simulink model "LR_5_var2"  (R2020b)
settings: Solver=VariableStepAuto  StartTime=0.0  StopTime=5  FixedStep=1e-4  RelTol=1e-3
values from neighbouring files (symbols this model uses):
  a = 0.2    [LR_5_param_var2.m]
  b = 1.5    [LR_5_param_var2.m]
  c1 = 4    [LR_5_param_var2.m]
  U = 3    [LR_5_param_var2.m]
  w = 10    [LR_5_param_var2.m]
libraries: simulink x17, powerlib_meascontrol x6
settings Model: SimulationMode=accelerator  Creator=SIA  LastModifiedBy=SIA
settings SolverCC: ZeroCrossAlgorithm=Adaptive  AlgebraicLoopSolver=LineSearch
settings DebuggingCC: IgnoredZcDiagnostic=none

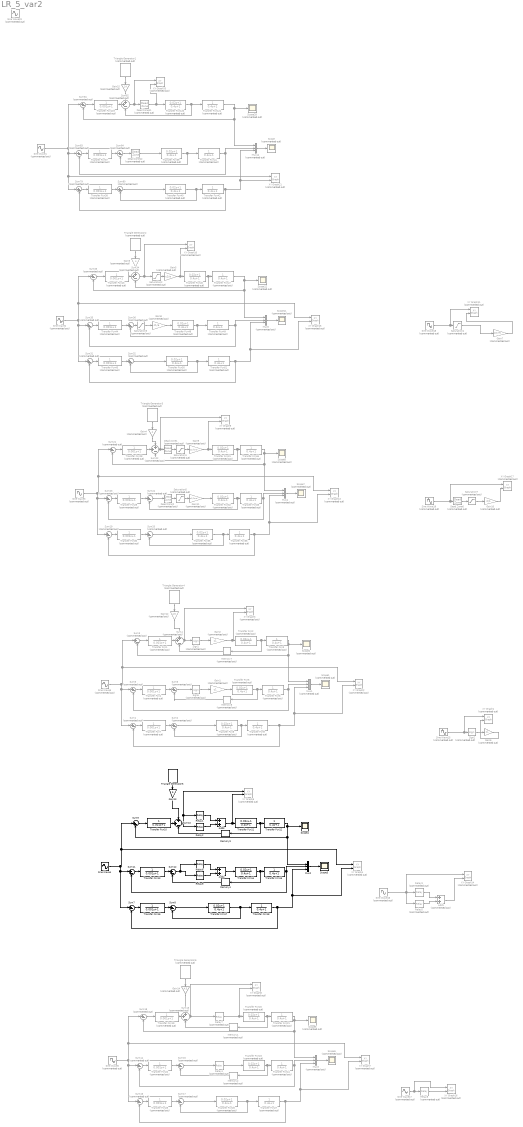
== system LR_5_var2 ==
  Add1 : Sum  Commented=on
  Add3 : Sum
  Add4 : Sum
  Dead Zone{1..2,11..12} (4 alike) : DeadZone  Commented=on  LowerValue=-a  UpperValue=a  SaturateOnIntegerOverflow=on
  Dead Zone6 : DeadZone  Commented=on  LowerValue=-1  UpperValue=1  SaturateOnIntegerOverflow=on
  Gain1 : Gain  Commented=on  Gain=c1
  Gain10 : Gain  Commented=on  Gain=2/1
  Gain11 : Gain  Commented=on  Gain=c1/(b-a)
  Gain12 : Gain  Commented=on  Gain=4.5
  Gain13 : Gain  Gain=5
  Gain14 : Gain  Commented=on  Gain=4.5
  Gain15 : Gain  Commented=on  Gain=14
  Gain2 : Gain  Commented=on  Gain=c1
  Gain3 : Gain  Commented=on  Gain=4
  Gain4 : Gain  Commented=on  Gain=4
  Gain5 : Gain  Commented=on  Gain=c1/a
  Gain6 : Gain  Commented=on  Gain=c1
  Gain7 : Gain  Commented=on  Gain=2/0.75
  Gain8 : Gain  Commented=on  Gain=c1/a
  Gain9 : Gain  Commented=on  Gain=c1/(b-a)
  Memory{1..2,7..8} (4 alike) : Memory  Commented=on
  Memory3 : Memory
  Memory4 : Memory
  Mux{1,3..4,6,14} (5 alike) : Mux  Commented=on  Inputs=3
  Mux2 : Mux  Inputs=3
  Relay1 : Relay  OnSwitchValue=a  OffSwitchValue=a  OnOutputValue=c1
  Relay2 : Relay  OnSwitchValue=-a  OffSwitchValue=-a  OnOutputValue=0  OffOutputValue=-c1
  Relay3 : Relay  Commented=on  OnSwitchValue=a  OffSwitchValue=a  OnOutputValue=c1
  Relay4 : Relay  Commented=on  OnSwitchValue=a  OffSwitchValue=-a  OnOutputValue=c1  OffOutputValue=-c1
  Relay5 : Relay  Commented=on  OnSwitchValue=-a  OffSwitchValue=-a  OnOutputValue=0  OffOutputValue=-c1
  Relay6 : Relay  OnSwitchValue=a  OffSwitchValue=a  OnOutputValue=c1
  Relay7 : Relay  Commented=on  OnSwitchValue=a  OffSwitchValue=-a  OnOutputValue=c1  OffOutputValue=-c1
  Relay8 : Relay  Commented=on  OnSwitchValue=a  OffSwitchValue=-a  OnOutputValue=c1  OffOutputValue=-c1
  Relay9 : Relay  OnSwitchValue=-a  OffSwitchValue=-a  OnOutputValue=0  OffOutputValue=-c1
  Saturation1 : Saturate  Commented=on  UpperLimit=b-a  LowerLimit=-(b-a)
  Saturation2 : Saturate  Commented=on  UpperLimit=a  LowerLimit=-a
  Saturation3 : Saturate  Commented=on  UpperLimit=a  LowerLimit=-a
  Saturation4 : Saturate  Commented=on  UpperLimit=0.75  LowerLimit=-0.75
  Saturation5 : Saturate  Commented=on  UpperLimit=b-a  LowerLimit=-(b-a)
  Saturation7 : Saturate  Commented=on  UpperLimit=1  LowerLimit=-1
  Scope{,1..2,5..8,11..12,28} (10 alike) : Scope  Commented=on
  Scope3 : Scope
  Scope4 : Scope
  Sign1 : Signum  Commented=on
  Sign2 : Signum  Commented=on
  Sign5 : Signum  Commented=on
  Sine Wave{1..3,5..6} (5 alike) : Sin  Commented=on  Amplitude=U  Frequency=w  SampleTime=0
  Sine Wave15 : Sin  Commented=on  Amplitude=3  Frequency=10  SampleTime=0
  Sine Wave16 : Sin  Commented=on  Amplitude=3  Phase=90  SampleTime=0
  Sine Wave17 : Sin  Commented=on  Amplitude=10  SampleTime=0
  Sine Wave18 : Sin  Commented=on  Amplitude=3  SampleTime=0
  Sine Wave19 : Sin  Commented=on  Amplitude=5  SampleTime=0
  Sine Wave23 : Sin  Commented=on  Amplitude=6  Frequency=1000  SampleTime=0
  Sine Wave4 : Sin  Amplitude=U  Frequency=w  SampleTime=0
  Sum{1..3,5..6,14..21,23..24,31..33,35..36,79..81,83..84} (25 alike) : Sum  Commented=on  Inputs=|+-
  Sum10 : Sum  Inputs=++-
  Sum{7..9,11..12} (5 alike) : Sum  Inputs=|+-
  Sum{4,13,22,34,82} (5 alike) : Sum  Commented=on  Inputs=++-
  Transfer Fcn{1,4,7,19,22,25,28..30,37..38,43..45,119} (15 alike) : TransferFcn  Commented=on  Denominator=[0.001 1]
  Transfer Fcn10 : TransferFcn  Denominator=[0.001 1]
  Transfer Fcn11 : TransferFcn  Numerator=[0.02 1]  Denominator=[0.4 1]
  Transfer Fcn12 : TransferFcn  Denominator=[0.4 1]
  Transfer Fcn{2,5,8,20,23,26,31..32,35,39..40,46,48,50,120} (15 alike) : TransferFcn  Commented=on  Numerator=[0.02 1]  Denominator=[0.4 1]
  Transfer Fcn{3,6,9,21,24,27,33..34,36,41..42,47,49,51,121} (15 alike) : TransferFcn  Commented=on  Denominator=[0.4 1]
  Transfer Fcn13 : TransferFcn  Denominator=[0.001 1]
  Transfer Fcn14 : TransferFcn  Numerator=[0.02 1]  Denominator=[0.4 1]
  Transfer Fcn15 : TransferFcn  Denominator=[0.4 1]
  Transfer Fcn16 : TransferFcn  Denominator=[0.001 1]
  Transfer Fcn17 : TransferFcn  Numerator=[0.02 1]  Denominator=[0.4 1]
  Transfer Fcn18 : TransferFcn  Denominator=[0.4 1]
  Triangle Generator{1..4} (4 alike) : powerlib_meascontrol/Pulse & Signal Generators/Triangle Generator  Commented=on  Freq=159.15494327  Phase=0  Ts=0
  Triangle Generator5 : powerlib_meascontrol/Pulse & Signal Generators/Triangle Generator  Freq=159.15494327  Phase=0  Ts=0
  Triangle Generator6 : powerlib_meascontrol/Pulse & Signal Generators/Triangle Generator  Commented=on  Freq=1590.15494327  Phase=0  Ts=0
  XY Graph1 : simulink/Sinks/XY Graph  Commented=on  xmin=-1  xmax=1  ymin=-4  ymax=4  st=0.001
  XY Graph10 : simulink/Sinks/XY Graph  Commented=on  xmin=-2  xmax=2  ymin=-4  ymax=4  st=-1
  XY Graph11 : simulink/Sinks/XY Graph  Commented=on  xmin=-1  xmax=1  ymin=-2  ymax=2  st=0.001
  XY Graph{2,4,7,13} (4 alike) : simulink/Sinks/XY Graph  Commented=on  xmin=-3  xmax=3  ymin=-0.5  ymax=0.5  st=0
  XY Graph14 : simulink/Sinks/XY Graph  Commented=on  xmin=-2  xmax=2  ymin=-4  ymax=4  st=0.001
  XY Graph15 : simulink/Sinks/XY Graph  Commented=on  xmin=-10  xmax=10  ymin=-0.3  ymax=0.3  st=0
  XY Graph16 : simulink/Sinks/XY Graph  Commented=on  xmin=-2  xmax=2  ymin=-4  ymax=4  st=0.001
  XY Graph17 : simulink/Sinks/XY Graph  Commented=on  xmin=-4  xmax=4  ymin=-2  ymax=2  st=0.001
  XY Graph20 : simulink/Sinks/XY Graph  Commented=on  xmin=-2  xmax=2  ymin=-1  ymax=1  st=-1
  XY Graph21 : simulink/Sinks/XY Graph  Commented=on  xmin=-10  xmax=10  ymin=-0.3  ymax=0.3  st=0
  XY Graph3 : simulink/Sinks/XY Graph  Commented=on  xmin=-2  xmax=2  ymin=-3  ymax=3  st=-1
  XY Graph6 : simulink/Sinks/XY Graph  Commented=on  xmin=-2  xmax=2  ymin=-3  ymax=3  st=-1
  XY Graph8 : simulink/Sinks/XY Graph  Commented=on  xmin=-2  xmax=2  ymin=-3  ymax=3  st=-1
  XY Graph9 : simulink/Sinks/XY Graph  Commented=on  xmin=-2  xmax=2  ymin=-4  ymax=4  st=-1
  wires:
  Sine Wave15/1 -> XY Graph1/1, Sign2/1
  Sign2/1 -> Gain6/1
  Gain6/1 -> XY Graph1/2
  Sine Wave16/1 -> Relay5/1, Relay3/1, XY Graph14/1
  Sine Wave17/1 -> Relay8/1, XY Graph16/1
  Relay8/1 -> XY Graph16/2
  Gain7/1 -> XY Graph11/2
  Sine Wave18/1 -> Saturation4/1, XY Graph11/1
  Saturation4/1 -> Gain7/1
  Sine Wave19/1 -> Dead Zone6/1, XY Graph17/1
  Gain10/1 -> XY Graph17/2
  Saturation7/1 -> Gain10/1
  Dead Zone6/1 -> Saturation7/1
  Transfer Fcn42/1 -> XY Graph21/2, Mux14/3, Sum79/2
  Transfer Fcn40/1 -> Transfer Fcn42/1, Sum80/2
  Sum80/1 -> Transfer Fcn40/1
  Dead Zone12/1 -> Transfer Fcn39/1
  Transfer Fcn39/1 -> Transfer Fcn41/1, Sum84/2
  Transfer Fcn121/1 -> Scope28/1, Mux14/1, Sum81/2
  Transfer Fcn41/1 -> Sum83/2, Mux14/2
  Transfer Fcn119/1 -> Sum82/2
  Sum82/1 -> XY Graph20/1, Dead Zone11/1
  Transfer Fcn37/1 -> Sum84/1
  Sum81/1 -> Transfer Fcn119/1
  Transfer Fcn38/1 -> Sum80/1
  Sum84/1 -> Dead Zone12/1
  Mux14/1 -> Scope/1
  Sum83/1 -> Transfer Fcn37/1
  Transfer Fcn120/1 -> Sum82/3, Transfer Fcn121/1
  Dead Zone11/1 -> XY Graph20/2, Transfer Fcn120/1
  Sum79/1 -> Transfer Fcn38/1
  Sine Wave1/1 -> Sum81/1, Sum79/1, XY Graph21/1, Sum83/1
  Transfer Fcn44/1 -> Sum36/1
  Sum35/1 -> Transfer Fcn44/1
  Saturation3/1 -> Gain8/1
  Transfer Fcn50/1 -> Transfer Fcn51/1, Sum32/2
  Transfer Fcn47/1 -> Scope12/1, Mux6/1, Sum33/2
  Transfer Fcn46/1 -> Transfer Fcn47/1, Sum34/3
  Saturation2/1 -> Gain5/1
  Transfer Fcn48/1 -> Transfer Fcn49/1, Sum36/2
  Sum31/1 -> Transfer Fcn45/1
  Sine Wave2/1 -> Sum33/1, XY Graph15/1, Sum31/1, Sum35/1
  Sum32/1 -> Transfer Fcn50/1
  Sum36/1 -> Saturation3/1
  Sum33/1 -> Transfer Fcn43/1
  Sum34/1 -> Saturation2/1, XY Graph10/1
  Mux6/1 -> Scope11/1
  Transfer Fcn43/1 -> Sum34/2
  Transfer Fcn51/1 -> XY Graph15/2, Mux6/3, Sum31/2
  Transfer Fcn45/1 -> Sum32/1
  Transfer Fcn49/1 -> Sum35/2, Mux6/2
  Gain5/1 -> Transfer Fcn46/1, XY Graph10/2
  Gain8/1 -> Transfer Fcn48/1
  Gain11/1 -> Transfer Fcn32/1
  Transfer Fcn34/1 -> Scope8/1, Mux4/1, Sum21/2
  Transfer Fcn29/1 -> Sum24/1
  Sum23/1 -> Transfer Fcn29/1
  Sum19/1 -> Transfer Fcn30/1
  Transfer Fcn32/1 -> Transfer Fcn33/1, Sum24/2
  Transfer Fcn31/1 -> Transfer Fcn34/1, Sum22/3
  Sine Wave3/1 -> Sum21/1, XY Graph13/1, Sum19/1, Sum23/1
  Sum20/1 -> Transfer Fcn35/1
  Gain9/1 -> Transfer Fcn31/1, XY Graph9/2
  Transfer Fcn33/1 -> Sum23/2, Mux4/2
  Transfer Fcn35/1 -> Transfer Fcn36/1, Sum20/2
  Transfer Fcn36/1 -> XY Graph13/2, Mux4/3, Sum19/2
  Mux4/1 -> Scope7/1
  Sum22/1 -> Dead Zone1/1, XY Graph9/1
  Transfer Fcn30/1 -> Sum20/1
  Transfer Fcn28/1 -> Sum22/2
  Gain4/1 -> Sum22/1
  Sum24/1 -> Dead Zone2/1
  Sum21/1 -> Transfer Fcn28/1
  Dead Zone2/1 -> Saturation5/1
  Saturation5/1 -> Gain11/1
  Gain2/1 -> XY Graph3/2, Transfer Fcn2/1
  Transfer Fcn1/1 -> Sum4/2
  Transfer Fcn7/1 -> Sum2/1
  Sum4/1 -> Sign1/1, XY Graph3/1
  Sum3/1 -> Transfer Fcn1/1
  Mux1/1 -> Scope1/1
  Transfer Fcn9/1 -> XY Graph2/2, Mux1/3, Sum1/2
  Transfer Fcn6/1 -> Sum5/2, Mux1/2
  Sum2/1 -> Transfer Fcn8/1
  Transfer Fcn5/1 -> Transfer Fcn6/1, Memory8/1
  Transfer Fcn2/1 -> Transfer Fcn3/1, Memory7/1
  Transfer Fcn4/1 -> Sum6/1
  Sum1/1 -> Transfer Fcn7/1
  Transfer Fcn8/1 -> Transfer Fcn9/1, Sum2/2
  Sum5/1 -> Transfer Fcn4/1
  Gain1/1 -> Transfer Fcn5/1
  Sine Wave5/1 -> Sum3/1, XY Graph2/1, Sum1/1, Sum5/1
  Sum6/1 -> Sign5/1
  Transfer Fcn3/1 -> Scope2/1, Mux1/1, Sum3/2
  Sign1/1 -> Gain2/1
  Sign5/1 -> Gain1/1
  Memory7/1 -> Sum4/3
  Memory8/1 -> Sum6/2
  Add3/1 -> Transfer Fcn11/1, XY Graph6/2
  Sum9/1 -> Transfer Fcn10/1
  Transfer Fcn16/1 -> Sum8/1
  Memory4/1 -> Sum12/2
  Transfer Fcn14/1 -> Transfer Fcn15/1, Memory4/1
  Sum8/1 -> Transfer Fcn17/1
  Transfer Fcn10/1 -> Sum10/2
  Transfer Fcn13/1 -> Sum12/1
  Transfer Fcn18/1 -> XY Graph4/2, Mux2/3, Sum7/2
  Sine Wave4/1 -> Sum9/1, XY Graph4/1, Sum7/1, Sum11/1
  Mux2/1 -> Scope3/1
  Transfer Fcn12/1 -> Scope4/1, Mux2/1, Sum9/2
  Transfer Fcn11/1 -> Memory3/1, Transfer Fcn12/1
  Memory3/1 -> Sum10/3
  Sum11/1 -> Transfer Fcn13/1
  Transfer Fcn15/1 -> Sum11/2, Mux2/2
  Transfer Fcn17/1 -> Transfer Fcn18/1, Sum8/2
  Sum7/1 -> Transfer Fcn16/1
  Sum10/1 -> Relay2/1, Relay1/1, XY Graph6/1
  Relay1/1 -> Add3/1
  Relay2/1 -> Add3/2
  Sum12/1 -> Relay6/1, Relay9/1
  Relay9/1 -> Add4/2
  Relay6/1 -> Add4/1
  Add4/1 -> Transfer Fcn14/1
  Relay5/1 -> Add1/2
  Relay3/1 -> Add1/1
  Add1/1 -> XY Graph14/2
  Memory1/1 -> Sum13/3
  Sum16/1 -> Transfer Fcn25/1
  Transfer Fcn26/1 -> Transfer Fcn27/1, Sum17/2
  Transfer Fcn24/1 -> Sum14/2, Mux3/2
  Relay7/1 -> Transfer Fcn20/1, XY Graph8/2
  Transfer Fcn23/1 -> Transfer Fcn24/1, Memory2/1
  Sum14/1 -> Transfer Fcn22/1
  Memory2/1 -> Sum15/2
  Sum13/1 -> Relay7/1, XY Graph8/1
  Sum18/1 -> Transfer Fcn19/1
  Sine Wave6/1 -> Sum18/1, XY Graph7/1, Sum16/1, Sum14/1
  Transfer Fcn21/1 -> Scope6/1, Mux3/1, Sum18/2
  Transfer Fcn20/1 -> Memory1/1, Transfer Fcn21/1
  Mux3/1 -> Scope5/1
  Sum15/1 -> Relay4/1
  Transfer Fcn27/1 -> XY Graph7/2, Mux3/3, Sum16/2
  Transfer Fcn19/1 -> Sum13/2
  Sum17/1 -> Transfer Fcn26/1
  Transfer Fcn25/1 -> Sum17/1
  Transfer Fcn22/1 -> Sum15/1
  Relay4/1 -> Transfer Fcn23/1
  Triangle Generator1/1 -> Gain15/1
  Gain15/1 -> Sum82/1
  Triangle Generator2/1 -> Gain3/1
  Triangle Generator3/1 -> Gain4/1
  Dead Zone1/1 -> Saturation1/1
  Saturation1/1 -> Gain9/1
  Triangle Generator4/1 -> Gain12/1
  Gain12/1 -> Sum4/1
  Gain13/1 -> Sum10/1
  Triangle Generator5/1 -> Gain13/1
  Gain3/1 -> Sum34/1
  Triangle Generator6/1 -> Gain14/1
  Gain14/1 -> Sum13/1
